simulink model "CONTROL_INVERSE_DYNAMICS"  (R2025b)
settings: Solver=VariableStepAuto  StartTime=0.0  StopTime=10.0  RelTol=1e-3
libraries: SCR x3
settings Model: Creator=Michael  LastModifiedBy=Michael

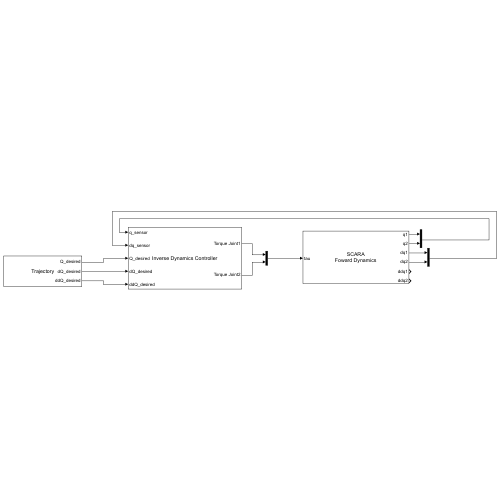
[thumbnail: Simulink's stored preview of the top-level diagram]
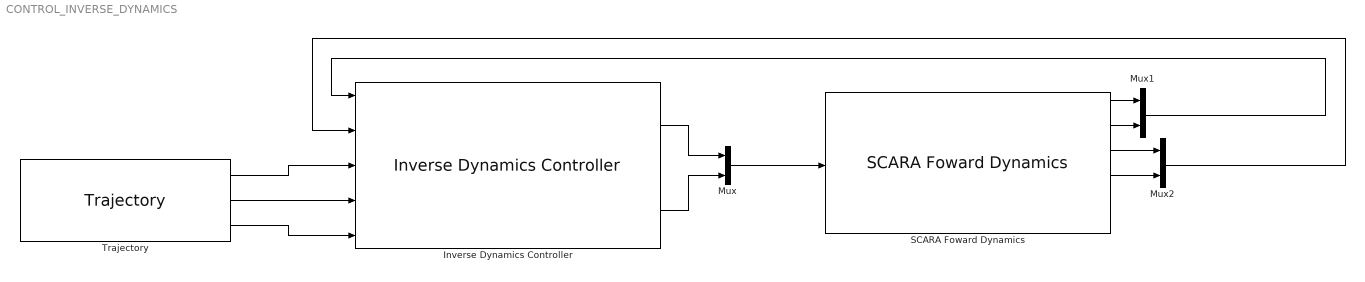
== system CONTROL_INVERSE_DYNAMICS ==
  Inverse Dynamics Controller : SCR/Inverse Dynamics Controller  SystemSampleTime=-1  VariantActivationTime=update diagram  EmptyChoice=off  PassThrough=off  PassThroughVariantControl=(default)  EmptyChoiceVariantControl=(default)  AllowFlexibleInterface=on  Latency=0  AutoFrameSizeCalculation=off
  Mux : Mux  Inputs=2
  Mux1 : Mux  Inputs=2
  Mux2 : Mux  Inputs=2
  SCARA Foward Dynamics : SCR/SCARA Foward Dynamics  SystemSampleTime=-1  VariantActivationTime=update diagram  EmptyChoice=off  PassThrough=off  PassThroughVariantControl=(default)  EmptyChoiceVariantControl=(default)  AllowFlexibleInterface=on  Latency=0  AutoFrameSizeCalculation=off
  Trajectory : SCR/Trajectory  SystemSampleTime=-1  VariantActivationTime=update diagram  EmptyChoice=off  PassThrough=off  PassThroughVariantControl=(default)  EmptyChoiceVariantControl=(default)  AllowFlexibleInterface=on  Latency=0  AutoFrameSizeCalculation=off
  wires:
  Trajectory/1 -> Inverse Dynamics Controller/3
  Trajectory/2 -> Inverse Dynamics Controller/4
  Trajectory/3 -> Inverse Dynamics Controller/5
  Mux/1 -> SCARA Foward Dynamics/1
  Mux1/1 -> Inverse Dynamics Controller/1
  Mux2/1 -> Inverse Dynamics Controller/2
  Inverse Dynamics Controller/2 -> Mux/2
  Inverse Dynamics Controller/1 -> Mux/1
  SCARA Foward Dynamics/1 -> Mux1/1
  SCARA Foward Dynamics/2 -> Mux1/2
  SCARA Foward Dynamics/3 -> Mux2/1
  SCARA Foward Dynamics/4 -> Mux2/2
